simulink model "AOCS_FDIR"  (R2020a)
settings: Solver=ode45  StartTime=0.0  StopTime=86400  FixedStep=1e-4  MaxStep=0.1  RelTol=1e-3  AbsTol=1e-3
undefined symbols (not defined in the file or in its folder): A, A_FEEP, A_FEEP_real, A_mag, CG_real, d_face, Dipole_SC, e0_0, e1_0, e2_0, e3_0, e_max_att, e_max_orb, Env_Drag, Env_J2, Env_Moon, Env_Sun, Env_TGG, Env_TMag, FEEP, g, GNSS, gyr, h_ref, h_RW, h_rw_0, I, I_real, IAU, initial_date_JD, J2, K_det, k_quat, km, m, mag, mu, mu_Moon, mu_Sun, n, n_orbits, q_0, Re, RW1, RW2, RW3, RW4, rx0, ry0, rz0, s, sigma1, sigma2, star, T_friction, th_2_gyr, th_FR_gyr, th_RW, th_SD_gyr_null, th_thruster ... (+10)
libraries: dspstat3 x16, aerolibutil x8, sharedutil x6, sharedtransform x5, vrlib x3, aerolibtransform2 x3, aerolibcelestial x2, aerolibgravity2 x1, dspinverses x1
(part 3 of 3)

== matlab function AOCS_FDIR/Navigation/Orbit Filter/MATLAB Function ==
  data: z input; rk1 output; dt input; sig_r input; sig_v input; vk1 output
function [rk1, vk1]  = Kalman(z, dt, sig_r, sig_v)

persistent xk Pk;

%% State transition matrix
A = [1 0 0 dt 0 0; 
     0 1 0 0 dt 0; 
     0 0 1 0 0 dt; 
     0 0 0 1 0 0; 
     0 0 0 0 1 0; 
     0 0 0 0 0 1];
 
%% Process noise matrix 
G = [dt^2/2 0      0;
     0      dt^2/2 0;
     0      0      dt^2/2;
     dt     0      0;
     0      dt     0;
     0      0      dt];
 
Q = 0.25^2*(G*G');
 
%% Sensor noise covariance matrix
R = [sig_r(1)^2 0 0 0 0 0;
     0 sig_r(2)^2 0 0 0 0;
     0 0 sig_r(3)^2 0 0 0;
     0 0 0 sig_v(1)^2 0 0;
     0 0 0 0 sig_v(2)^2 0;
     0 0 0 0 0 sig_v(3)^2];
 
%% Initialize States and Measurement
if isempty(xk)
    % Initialize states
    xk = z;
    
    % Initialize Covariance Matrix. Farrenkopf’s steady-state analysis
    Pk = R;
    
    % Initialize Measurement
    xk1    = xk;
    rk1 = xk1(1:3);
    vk1 = xk1(4:6);
    
    return;
end

%% Prediction
xk1 = A*xk;
Pk1 = A*Pk*A'+Q;

%% Correction
K   = Pk1/(Pk1+R);
xk1 = xk1 + K*(z-xk1);
Pk1 = (eye(6)-K)*Pk1;

rk1 = xk1(1:3);
vk1 = xk1(4:6);

%% Update
xk = xk1;
Pk = Pk1;

return

== matlab function AOCS_FDIR/Control/Attitude Control/Reaction Wheel Model/Desaturation/MATLAB Function1 ==
  data: us input; T_det output; T_mt input; A_rw input
function T_det = fcn(us, T_mt, A_rw)

delta_u = (A_rw'/(A_rw*A_rw'))*(T_mt-A_rw*us);
T_det   = delta_u;

== matlab function AOCS_FDIR/Navigation/Gyroscope/Gyroscope Model/Artificial Failure/MATLAB Function2 ==
  settings: updateMethod=DISCRETE
  data: t input; flag1 input; flag2 input; flag3 input; in input; out output
function out = fcn(t, flag1, flag2, flag3,in)

persistent frozen
persistent t0

drift = 1e-6;

if isempty(frozen)
    frozen=0;
end

if isempty(t0)
    t0=0;
end

if flag1>0
%% Sudden Death
    out = 0;
elseif flag2>0
%% Frozen Signal
    if frozen == 0
        frozen=in;
        out = in;
    else
        out = frozen;
    end
elseif flag3>0
    %% Drift x
    if t0 == 0
        t0=t;
        out = in;
    else
        out = in + drift*1.37*(t-t0);
    end
else
    out = in;
    frozen = 0;
    t0 = 0;
end

== matlab function AOCS_FDIR/FDIR/Gyroscopes FDIR/Level 1/Diagnosis Frozen Signal/MATLAB Function ==
  settings: updateMethod=DISCRETE
  data: std_1 input; flag_FR_1 output; std_2 input; std_3 input; std_4 input; std_5 input; std_6 input; th_FR_gyr input; win_length input; gyr_rate input; t input; flag_FR_2 output; flag_FR_3 output; flag_FR_4 output; flag_FR_5 output; flag_FR_6 output
function [flag_FR_1,flag_FR_2,flag_FR_3,flag_FR_4,flag_FR_5,flag_FR_6] = fcn(std_1,std_2,std_3,std_4,std_5,std_6,th_FR_gyr, win_length, gyr_rate, t)
%% Define persistent variables
persistent flag1
persistent flag2
persistent flag3
persistent flag4
persistent flag5
persistent flag6

if isempty(flag1)
    flag1 = 0;
end

if isempty(flag2)
    flag2 = 0;
end

if isempty(flag3)
    flag3 = 0;
end

if isempty(flag4)
    flag4 = 0;
end

if isempty(flag5)
    flag5 = 0;
end

if isempty(flag6)
    flag6 = 0;
end

%% Wait to moving std stabilization
if t<win_length*gyr_rate
    flag_FR_1 = flag1;
    flag_FR_2 = flag2;
    flag_FR_3 = flag3;
    flag_FR_4 = flag4;
    flag_FR_5 = flag5;
    flag_FR_6 = flag6;
    return
end

%% Detect the Frozen Condition
if std_1<th_FR_gyr
    flag1 = 1;   
end

if std_2<th_FR_gyr
    flag2 = 1;   
end

if std_3<th_FR_gyr
    flag3 = 1;   
end

if std_4<th_FR_gyr
    flag4 = 1;   
end

if std_5<th_FR_gyr
    flag5 = 1;   
end

if std_6<th_FR_gyr
    flag6 = 1;   
end

%% Create the output
flag_FR_1 = flag1;
flag_FR_2 = flag2;
flag_FR_3 = flag3;
flag_FR_4 = flag4;
flag_FR_5 = flag5;
flag_FR_6 = flag6;

== matlab function AOCS_FDIR/FDIR/Gyroscopes FDIR/Level 1/MATLAB Function ==
  data: flag_SD input; flagLevel1 output; flag_FR input
function flagLevel1 = fcn(flag_SD, flag_FR)
%% Define persistent variables
persistent flag

if isempty(flag)
    flag = zeros(6,1);
end

%% Detect the failure
if flag_SD(1)>0 || flag_FR(1)>0
    flag(1) = 1;
end

if flag_SD(2)>0 || flag_FR(2)>0
    flag(2) = 1;
end

if flag_SD(3)>0 || flag_FR(3)>0
    flag(3) = 1;
end

if flag_SD(4)>0 || flag_FR(4)>0
    flag(4) = 1;
end

if flag_SD(5)>0 || flag_FR(5)>0
    flag(5) = 1;
end

if flag_SD(6)>0 || flag_FR(6)>0
    flag(6) = 1;
end

%% Create the output
flagLevel1 = flag;

== matlab function AOCS_FDIR/Navigation/Gyroscope/Gyroscope Model/Gyroscope Recovery ==
  data: H_in input; H_out output; flagLevel1 input; flagLevel2 input
function H_out = fcn(H_in,flagLevel1,flagLevel2)
%% Switch off (=0) the faulty gyroscopes
% Number 1
if flagLevel1(1) == 0
    if flagLevel2(1) == 0
        switch_m1 = 1;
    else
        switch_m1 = 0;
    end
else
    switch_m1 = 0;
end

% Number 2
if flagLevel1(2) == 0
    if flagLevel2(2) == 0
        switch_m2 = 1;
    else
        switch_m2 = 0;
    end
else
    switch_m2 = 0;
end

% Number 3
if flagLevel1(3) == 0
    if flagLevel2(3) == 0
        switch_m3 = 1;
    else
        switch_m3 = 0;
    end
else
    switch_m3 = 0;
end

% Number 4
if flagLevel1(4) == 0
    if flagLevel2(4) == 0
        switch_m4 = 1;
    else
        switch_m4 = 0;
    end
else
    switch_m4 = 0;
end

% Number 5
if flagLevel1(5) == 0
    if flagLevel2(5) == 0
        switch_m5 = 1;
    else
        switch_m5 = 0;
    end
else
    switch_m5 = 0;
end

% Number 6
if flagLevel1(6) == 0
    if flagLevel2(6) == 0
        switch_m6 = 1;
    else
        switch_m6 = 0;
    end
else
    switch_m6 = 0;
end

%% Final configuration matrix
H_out = [H_in(1,:)*switch_m1;
         H_in(2,:)*switch_m2;
         H_in(3,:)*switch_m3;
         H_in(4,:)*switch_m4;
         H_in(5,:)*switch_m5;
         H_in(6,:)*switch_m6];

== matlab function AOCS_FDIR/Control/Attitude Control/Reaction Wheel Model/Artificial Failure1/MATLAB Function ==
  settings: updateMethod=DISCRETE
  data: in input; h_RW input; T_friction input; out output; flag1 input; flag2 input; flag3 input
function out = fcn(in, h_RW, T_friction, flag1, flag2, flag3)

if flag1>0
%% Motor failure
    out = T_friction*sign(h_RW);
elseif flag2>0
%% Friction failure
    out = in*0.75;
elseif flag3>0
%% Loss of accuracy
    out = in*(1-0.3*randn);
else
    out = in;
end

== matlab function AOCS_FDIR/Navigation/Gyroscope/Gyroscope Model/Isolation Switch off  ==
  data: in input; out output; flagLevel1 input; flagLevel2 input
function out = fcn(in, flagLevel1, flagLevel2)
%% The signal from the faulty gyroscopes must be null
% Number 1
if flagLevel1(1) == 0
    if flagLevel2(1) == 0
        switch_m1 = 1;
    else
        switch_m1 = 0;
    end
else
    switch_m1 = 0;
end

% Number 2
if flagLevel1(2) == 0
    if flagLevel2(2) == 0
        switch_m2 = 1;
    else
        switch_m2 = 0;
    end
else
    switch_m2 = 0;
end

% Number 3
if flagLevel1(3) == 0
    if flagLevel2(3) == 0
        switch_m3 = 1;
    else
        switch_m3 = 0;
    end
else
    switch_m3 = 0;
end

% Number 4
if flagLevel1(4) == 0
    if flagLevel2(4) == 0
        switch_m4 = 1;
    else
        switch_m4 = 0;
    end
else
    switch_m4 = 0;
end

% Number 5
if flagLevel1(5) == 0
    if flagLevel2(5) == 0
        switch_m5 = 1;
    else
        switch_m5 = 0;
    end
else
    switch_m5 = 0;
end

% Number 6
if flagLevel1(6) == 0
    if flagLevel2(6) == 0
        switch_m6 = 1;
    else
        switch_m6 = 0;
    end
else
    switch_m6 = 0;
end

%% Compute output signal
out = [in(1)*switch_m1;
       in(2)*switch_m2;
       in(3)*switch_m3;
       in(4)*switch_m4;
       in(5)*switch_m5;
       in(6)*switch_m6];

== matlab function AOCS_FDIR/FDIR/Gyroscopes FDIR/Level 2/Fault Detection ==
  settings: updateMethod=DISCRETE
  data: flagr1 input; flagm1 output; flagr2 input; flagr3 input; flagr4 input; flagr5 input; flagr6 input; flagr7 input; flagr8 input; flagr9 input; flag input; flagm2 output; flagm3 output; flagm4 output; flagm5 output; flagm6 output
function [flagm1, flagm2, flagm3, flagm4, flagm5, flagm6] = fcn(flagr1, flagr2, flagr3, flagr4, flagr5, flagr6, flagr7, flagr8, flagr9,flag)
%% Define persistent variables
persistent flag1
persistent flag2
persistent flag3
persistent flag4
persistent flag5
persistent flag6

if isempty(flag1)
    flag1=0;
end

if isempty(flag2)
    flag2=0;
end

if isempty(flag3)
    flag3=0;
end

if isempty(flag4)
    flag4=0;
end

if isempty(flag5)
    flag5=0;
end

if isempty(flag6)
    flag6=0;
end

%% Failure dectection
if flag>0
    if flagr1 == 0
        if flagr2 ==1
            if flagr4 ==0
                flag6 = 1;
            elseif flagr4 ==1
                if flagr5 == 0
                    flag3 = 1;
                elseif flagr5 == 1
                    flag3 = 1;
                    flag6 = 1;
                end
            end
        end
    elseif flagr1 == 1
        if flagr2 == 0
            if flagr6 == 0
                flag4 = 1;
            elseif flagr6 == 1
                if flagr7 == 0
                    flag1 = 1;
                elseif flagr7 == 1
                    flag1 = 1;
                    flag4 = 1;
                end
            end
        elseif flagr2 == 1
            if flagr3 == 0
                if flagr4 == 0
                    flag2 = 1;
                elseif flagr4 == 1
                    if flagr5 == 0
                        flag5 = 1;
                    elseif flagr5 == 1
                        flag2 = 1;
                        flag5 = 1;
                    end
                end
            elseif flagr3 == 1
                if flagr7 == 0
                    flag1 = 1;
                    flag3 = 1;
                elseif flagr5 == 0
                    flag3 = 1;
                    flag5 = 1;
                elseif flagr6 == 0
                    flag4 = 1;
                    flag6 = 1;
                elseif flagr4 == 0
                    flag2 = 1;
                    flag6 = 1;
                elseif flagr9 == 0
                    flag1 = 1;
                    flag5 = 1;
                elseif flagr8 == 0
                    flag2 = 1;
                    flag4 = 1;
                end
            end
        end
    end
end


%% Assign the output
flagm1 = flag1;
flagm2 = flag2;
flagm3 = flag3;
flagm4 = flag4;
flagm5 = flag5;
flagm6 = flag6;

== matlab function AOCS_FDIR/Navigation/Gyroscope/Gyroscope Model/Artificial Failure/MATLAB Function1 ==
  settings: updateMethod=DISCRETE
  data: t input; flag1 input; flag2 input; flag3 input; in input; out output
function out = fcn(t, flag1, flag2, flag3,in)

persistent frozen
persistent t0

drift = 1e-6;

if isempty(frozen)
    frozen=0;
end

if isempty(t0)
    t0=0;
end

if flag1>0
%% Sudden Death
    out = 0;
elseif flag2>0
%% Frozen Signal
    if frozen == 0
        frozen=in;
        out = in;
    else
        out = frozen;
    end
elseif flag3>0
    %% Drift x
    if t0 == 0
        t0=t;
        out = in;
    else
        out = in + drift*1.15*(t-t0);
    end
else
    out = in;
    frozen = 0;
    t0 = 0;
end

== matlab function AOCS_FDIR/Control/Attitude Control/Reaction Wheel Model/Artificial Failure2/MATLAB Function ==
  settings: updateMethod=DISCRETE
  data: in input; h_RW input; T_friction input; out output; flag1 input; flag2 input; flag3 input
function out = fcn(in, h_RW, T_friction, flag1, flag2, flag3)

if flag1>0
%% Motor failure
    out = T_friction*sign(h_RW);
elseif flag2>0
%% Friction failure
    out = in*0.75;
elseif flag3>0
%% Loss of accuracy
    out = in*(1-0.3*randn);
else
    out = in;
end

== matlab function AOCS_FDIR/Control/Attitude Control/Reaction Wheel Model/Isolation2/MATLAB Function ==
  data: T_in input; T_out output; stop input; h_RW input; T_friction input; flagRW input
function T_out = fcn(T_in, stop, h_RW, T_friction, flagRW)

if flagRW>0
    if stop>0
        T_out = 0;
    else
        T_out = T_friction*sign(h_RW);
    end
else
    T_out = T_in;
end

== matlab function AOCS_FDIR/Control/Attitude Control/Reaction Wheel Model/Artificial Failure3/MATLAB Function ==
  settings: updateMethod=DISCRETE
  data: in input; h_RW input; T_friction input; out output; flag1 input; flag2 input; flag3 input
function out = fcn(in, h_RW, T_friction, flag1, flag2, flag3)

if flag1>0
%% Motor failure
    out = T_friction*sign(h_RW);
elseif flag2>0
%% Friction failure
    out = in*0.75;
elseif flag3>0
%% Loss of accuracy
    out = in*(1-0.3*randn);
else
    out = in;
end

== matlab function AOCS_FDIR/FDIR/Gyroscopes FDIR/Level 2/Residuals Generator ==
  data: w_gyr input; r1 output; r2 output; r3 output; r4 output; r5 output; r6 output; r7 output; r8 output; r9 output
function [r1,r2,r3,r4,r5,r6,r7,r8,r9] = fcn(w_gyr)
%% Measurements from gyroscopes
m1 = w_gyr(1);
m2 = w_gyr(2);
m3 = w_gyr(3);
m4 = w_gyr(4);
m5 = w_gyr(5);
m6 = w_gyr(6);

%% Residuals for detection
r1 = (m1+m4) - (m2+m5);
r2 = (m2+m5) - (m3+m6);
r3 = (m3+m6) - (m1+m4);

%% Residuals for isolation
r4 = 2*(m1+m3+m5) - 3*(m1+m4);
r5 = 2*(m2+m4+m6) - 3*(m1+m4);
r6 = 2*(m1+m3+m5) - 3*(m2+m5);
r7 = 2*(m2+m4+m6) - 3*(m2+m5);
r8 = 2*(m1+m3+m5) - 3*(m3+m6);
r9 = 2*(m2+m4+m6) - 3*(m3+m6);

== matlab function AOCS_FDIR/FDIR/Reaction Wheels FDIR/RW Diagnosis/Diagnosis Reaction Wheels ==
  settings: updateMethod=DISCRETE
  data: r_RW1 input; flagRW1 output; r_RW2 input; r_RW3 input; r_RW4 input; t input; RW_rate input; win_length input; flagRW2 output; flagRW3 output; flagRW4 output; th_RW input
function [flagRW1, flagRW2, flagRW3, flagRW4] = fcn(r_RW1, r_RW2, r_RW3, r_RW4, t, RW_rate, win_length,th_RW)

persistent flag

if t<2*win_length*RW_rate
    flagRW1 = 0;
    flagRW2 = 0;
    flagRW3 = 0;
    flagRW4 = 0;
    return
end

if isempty(flag)
    flag = zeros(4,1);
end

if r_RW1>th_RW
    flag(1) = 1;
end

if r_RW2>th_RW
    flag(2) = 1;
end

if r_RW3>th_RW
    flag(3) = 1;
end

if r_RW4>th_RW
    flag(4) = 1;
end

flagRW1 = flag(1);
flagRW2 = flag(2);
flagRW3 = flag(3);
flagRW4 = flag(4);

== matlab function AOCS_FDIR/Control/Attitude Control/Reaction Wheel Model/Isolation1/MATLAB Function ==
  data: T_in input; T_out output; stop input; h_RW input; T_friction input; flagRW input
function T_out = fcn(T_in, stop, h_RW, T_friction, flagRW)

if flagRW>0
    if stop>0
        T_out = 0;
    else
        T_out = T_friction*sign(h_RW);
    end
else
    T_out = T_in;
end

== matlab function AOCS_FDIR/Visualization/COE/MATLAB Function ==
  data: R input; a output; V input; e output; i output; RA output; w output; TA output
function [a, e, i, RA, w, TA] = sv2coe(R,V)
%-------------------------------------------------------------------------
% This function computes the classical orbital elements (coe)
% from the state vector (R,V).
%
% mu - gravitational parameter (mˆ3/sˆ2)
% R - position vector in ECI (m)
% V - velocity vector in ECI (m)
% r, v - the moduli of R and V
% vr - radial velocity component (m/s)
% H - the angular momentum vector (mˆ2/s)
% h - the moduli of H (mˆ2/s)
% i - inclination of the orbit (rad)
% N - the node line vector (mˆ2/s)
% n - the moduli of N
% cp - cross product of N and R
% RA - right ascension of the ascending node (rad)
% E - eccentricity vector
% e - eccentricity (moduli of E)
% eps - a small number below which the eccentricity is
% considered to be zero
% w - argument of perigee (rad)
% TA - true anomaly (rad)
% a - semimajor axis (m)
% coe - vector of orbital elements [a, e, i, RA, w, TA]
%
% ------------------------------------------------------------------------
%% Inputs
mu = 3.986004418e14;
eps = 1.e-10;

r = norm(R);
v = norm(V);
vr = dot(R,V)/r;

H = cross(R,V);
h = norm(H);

%% Inclination
i = acosd(H(3)/h);

%% Node line
N = cross([0 0 1],H);
n = norm(N);

%% Right Ascension
if n ~= 0
    RA = acosd(N(1)/n);
    if N(2) < 0
        RA = 360 - RA;
    end
else
    RA= 0;                 % No defined asceding node (Equatorial orbit)
end

%% Eccentricity
E = 1/mu*((v^2 - mu/r)*R - r*vr*V);
e = norm(E);

%% Argument of periapsis
% To avoid numerical errors
d_N_E=dot(N,E)/n/e;
if d_N_E>1 
    d_N_E = 1;
elseif d_N_E<-1
    d_N_E = -1;
end

if n ~= 0
    if e > eps
        w = acosd(d_N_E);
        if E(3) < 0
            w = 360 - w;
        end
    else
        w = 0;             % No defined periapsis (Circular orbit)    
    end
else
    w = 0;                 % No defined ascending node (Equatorial orbits)
end


%% True anomaly
% To avoid numerical errors
d_E_R=dot(E,R)/e/r;
if d_E_R>1 
    d_E_R = 1;
elseif d_E_R<-1
    d_E_R = -1;
end

d_N_R=dot(N,R)/n/r;
if d_N_R>1 
    d_N_R = 1;
elseif d_N_R<-1
    d_N_R = -1;
end

if e > eps
    TA = norm(acosd(d_E_R));
    if vr < 0
        TA = 360 - TA;
    end
else
    cp = cross(N,R);
    if cp(3) >= 0
        TA = acosd(d_N_R);
    else
        TA = 360 - acosd(d_N_R);
    end
end

%% Semimajor axis
a = h^2/mu/(1 - e^2);

== matlab function AOCS_FDIR/Control/Attitude Control/Reaction Wheel Allocation/Recovery ==
  data: RW1 input; A_rw output; RW2 input; RW3 input; RW4 input; flagRW1 input; flagRW2 input; flagRW3 input; flagRW4 input
function A_rw = fcn(RW1, RW2, RW3, RW4, flagRW1, flagRW2, flagRW3, flagRW4)
%% Switch off (=0) the faulty wheels
% Wheel 1
if flagRW1>0
    flag1 = 0;
else
    flag1 = 1;
end

% Wheel 2
if flagRW2>0
    flag2 = 0;
else
    flag2 = 1;
end

% Wheel 3
if flagRW3>0
    flag3 = 0;
else
    flag3 = 1;
end

% Wheel 4
if flagRW4>0
    flag4 = 0;
else
    flag4 = 1;
end

%% Reconfigure configuration matrix
A_rw = [RW1*flag1,RW2*flag2,RW3*flag3,RW4*flag4];

== matlab function AOCS_FDIR/Control/Attitude Control/Reaction Wheel Model/Desaturation/Recovery ==
  data: RW1 input; A_rw output; RW2 input; RW3 input; RW4 input; flagRW1 input; flagRW2 input; flagRW3 input; flagRW4 input
function A_rw = fcn(RW1, RW2, RW3, RW4, flagRW1, flagRW2, flagRW3, flagRW4)
%% Switch off (=0) the faulty wheels
% Wheel 1
if flagRW1>0
    flag1 = 0;
else
    flag1 = 1;
end

% Wheel 2
if flagRW2>0
    flag2 = 0;
else
    flag2 = 1;
end

% Wheel 3
if flagRW3>0
    flag3 = 0;
else
    flag3 = 1;
end

% Wheel 4
if flagRW4>0
    flag4 = 0;
else
    flag4 = 1;
end

%% Reconfigure configuration matrix
A_rw = [RW1*flag1,RW2*flag2,RW3*flag3,RW4*flag4];

== matlab function AOCS_FDIR/FDIR/Gyroscopes FDIR/Level 2/Evaluation ==
  data: S1 input; flagr1 output; S2 input; S3 input; S4 input; S5 input; S6 input; S7 input; S8 input; S9 input; win_length input; th input; flagr2 output; flagr3 output; flagr4 output; flagr5 output; flagr6 output; flagr7 output; flagr8 output; flagr9 output; flag output
function [flagr1, flagr2, flagr3, flagr4, flagr5, flagr6, flagr7,flagr8,flagr9,flag] = fcn(S1, S2, S3, S4, S5, S6, S7,S8,S9, win_length, th)
%% Define persistent variables
persistent state
persistent count

if isempty(count)
    state =zeros(9,2);
end

if isempty(count)
    count=0;
end

%% Evaluation of thresholds
if S1>th
    flagr1 = 1;
else
    flagr1 = 0;
end

if S2>th
    flagr2 = 1;
else
    flagr2 = 0;
end

if S3>th
    flagr3 = 1;
else
    flagr3 = 0;
end

if S4>th
    flagr4 = 1;
else
    flagr4 = 0;
end

if S5>th
    flagr5 = 1;
else
    flagr5 = 0;
end

if S6>th
    flagr6 = 1;
else
    flagr6 = 0;
end

if S7>th
    flagr7 = 1;
else
    flagr7 = 0;
end

if S8>th
    flagr8 = 1;
else
    flagr8 = 0;
end

if S9>th
    flagr9 = 1;
else
    flagr9 = 0;
end

%% Wait for stabilization of all residuals
for i=2
    state(:,i-1) = state(:,i);
end

state(1,2) = flagr1;
state(2,2) = flagr2;
state(3,2) = flagr3;
state(4,2) = flagr4;
state(5,2) = flagr5;
state(6,2) = flagr6;
state(7,2) = flagr7;
state(8,2) = flagr8;
state(9,2) = flagr9;

for i=1:9
    if state(i,1)~= state(i,2)
        count = 0;
    end
end

if flagr1>0 || flagr2>0 || flagr3>0
    count = count+1;
else
    count = 0;
end

if count>0.5*win_length
    flag = 1;
else
    flag =0;
end

== matlab function AOCS_FDIR/Navigation/Gyroscope/Gyroscope Model/Artificial Failure/MATLAB Function3 ==
  settings: updateMethod=DISCRETE
  data: t input; flag1 input; flag2 input; flag3 input; in input; out output
function out = fcn(t, flag1, flag2, flag3,in)

persistent frozen
persistent t0

drift = 1e-6;

if isempty(frozen)
    frozen=0;
end

if isempty(t0)
    t0=0;
end

if flag1>0
%% Sudden Death
    out = 0;
elseif flag2>0
%% Frozen Signal
    if frozen == 0
        frozen=in;
        out = in;
    else
        out = frozen;
    end
elseif flag3>0
    %% Drift x
    if t0 == 0
        t0=t;
        out = in;
    else
        out = in + drift*0.87*(t-t0);
    end
else
    out = in;
    frozen = 0;
    t0 = 0;
end

== matlab function AOCS_FDIR/Navigation/Gyroscope/Gyroscope Model/Artificial Failure/MATLAB Function4 ==
  settings: updateMethod=DISCRETE
  data: t input; flag1 input; flag2 input; flag3 input; in input; out output
function out = fcn(t, flag1, flag2, flag3,in)

persistent frozen
persistent t0

drift = 1e-6;

if isempty(frozen)
    frozen=0;
end

if isempty(t0)
    t0=0;
end

if flag1>0
%% Sudden Death
    out = 0;
elseif flag2>0
%% Frozen Signal
    if frozen == 0
        frozen=in;
        out = in;
    else
        out = frozen;
    end
elseif flag3>0
    %% Drift x
    if t0 == 0
        t0=t;
        out = in;
    else
        out = in + drift*(t-t0);
    end
else
    out = in;
    frozen = 0;
    t0 = 0;
end

== matlab function AOCS_FDIR/Navigation/Gyroscope/Gyroscope Model/Artificial Failure/MATLAB Function5 ==
  settings: updateMethod=DISCRETE
  data: t input; flag1 input; flag2 input; flag3 input; in input; out output
function out = fcn(t, flag1, flag2, flag3,in)

persistent frozen
persistent t0

drift = 1e-6;

if isempty(frozen)
    frozen=0;
end

if isempty(t0)
    t0=0;
end

if flag1>0
%% Sudden Death
    out = 0;
elseif flag2>0
%% Frozen Signal
    if frozen == 0
        frozen=in;
        out = in;
    else
        out = frozen;
    end
elseif flag3>0
    %% Drift x
    if t0 == 0
        t0=t;
        out = in;
    else
        out = in + drift*0.9*(t-t0);
    end
else
    out = in;
    frozen = 0;
    t0 = 0;
end

== matlab function AOCS_FDIR/Navigation/Gyroscope/Gyroscope Model/Artificial Failure/MATLAB Function6 ==
  settings: updateMethod=DISCRETE
  data: t input; flag1 input; flag2 input; flag3 input; in input; out output
function out = fcn(t, flag1, flag2, flag3,in)

persistent frozen
persistent t0

drift = 1e-6;

if isempty(frozen)
    frozen=0;
end

if isempty(t0)
    t0=0;
end

if flag1>0
%% Sudden Death
    out = 0;
elseif flag2>0
%% Frozen Signal
    if frozen == 0
        frozen=in;
        out = in;
    else
        out = frozen;
    end
elseif flag3>0
    %% Drift x
    if t0 == 0
        t0=t;
        out = in;
    else
        out = in + drift*0.66*(t-t0);
    end
else
    out = in;
    frozen = 0;
    t0 = 0;
end

== matlab function AOCS_FDIR/Control/Attitude Control/Reaction Wheel Model/Isolation3/MATLAB Function ==
  data: T_in input; T_out output; stop input; h_RW input; T_friction input; flagRW input
function T_out = fcn(T_in, stop, h_RW, T_friction, flagRW)

if flagRW>0
    if stop>0
        T_out = 0;
    else
        T_out = T_friction*sign(h_RW);
    end
else
    T_out = T_in;
end

== matlab function AOCS_FDIR/Control/Attitude Control/Reaction Wheel Model/Artificial Failure4/MATLAB Function ==
  settings: updateMethod=DISCRETE
  data: in input; h_RW input; T_friction input; out output; flag1 input; flag2 input; flag3 input
function out = fcn(in, h_RW, T_friction, flag1, flag2, flag3)

if flag1>0
%% Motor failure
    out = T_friction*sign(h_RW);
elseif flag2>0
%% Friction failure
    out = in*0.75;
elseif flag3>0
%% Loss of accuracy
    out = in*(1-0.3*randn);
else
    out = in;
end

== matlab function AOCS_FDIR/Control/Attitude Control/Reaction Wheel Model/Isolation4/MATLAB Function ==
  data: T_in input; T_out output; stop input; h_RW input; T_friction input; flagRW input
function T_out = fcn(T_in, stop, h_RW, T_friction, flagRW)

if flagRW>0
    if stop>0
        T_out = 0;
    else
        T_out = T_friction*sign(h_RW);
    end
else
    T_out = T_in;
end

== matlab function AOCS_FDIR/Visualization/COE/MATLAB Function1 ==
  data: R input; a output; V input; e output; i output; RA output; w output; TA output
function [a, e, i, RA, w, TA] = sv2coe(R,V)
%-------------------------------------------------------------------------
% This function computes the classical orbital elements (coe)
% from the state vector (R,V).
%
% mu - gravitational parameter (mˆ3/sˆ2)
% R - position vector in ECI (m)
% V - velocity vector in ECI (m)
% r, v - the moduli of R and V
% vr - radial velocity component (m/s)
% H - the angular momentum vector (mˆ2/s)
% h - the moduli of H (mˆ2/s)
% i - inclination of the orbit (rad)
% N - the node line vector (mˆ2/s)
% n - the moduli of N
% cp - cross product of N and R
% RA - right ascension of the ascending node (rad)
% E - eccentricity vector
% e - eccentricity (moduli of E)
% eps - a small number below which the eccentricity is
% considered to be zero
% w - argument of perigee (rad)
% TA - true anomaly (rad)
% a - semimajor axis (m)
% coe - vector of orbital elements [a, e, i, RA, w, TA]
%
% ------------------------------------------------------------------------
%% Inputs
mu = 3.986004418e14;
eps = 1.e-10;

r = norm(R);
v = norm(V);
vr = dot(R,V)/r;

H = cross(R,V);
h = norm(H);

%% Inclination
i = acosd(H(3)/h);

%% Node line
N = cross([0 0 1],H);
n = norm(N);

%% Right Ascension
if n ~= 0
    RA = acosd(N(1)/n);
    if N(2) < 0
        RA = 360 - RA;
    end
else
    RA= 0;                 % No defined asceding node (Equatorial orbit)
end

%% Eccentricity
E = 1/mu*((v^2 - mu/r)*R - r*vr*V);
e = norm(E);

%% Argument of periapsis
% To avoid numerical errors
d_N_E=dot(N,E)/n/e;
if d_N_E>1 
    d_N_E = 1;
elseif d_N_E<-1
    d_N_E = -1;
end

if n ~= 0
    if e > eps
        w = acosd(d_N_E);
        if E(3) < 0
            w = 360 - w;
        end
    else
        w = 0;             % No defined periapsis (Circular orbit)    
    end
else
    w = 0;                 % No defined ascending node (Equatorial orbits)
end


%% True anomaly
% To avoid numerical errors
d_E_R=dot(E,R)/e/r;
if d_E_R>1 
    d_E_R = 1;
elseif d_E_R<-1
    d_E_R = -1;
end

d_N_R=dot(N,R)/n/r;
if d_N_R>1 
    d_N_R = 1;
elseif d_N_R<-1
    d_N_R = -1;
end

if e > eps
    TA = norm(acosd(d_E_R));
    if vr < 0
        TA = 360 - TA;
    end
else
    cp = cross(N,R);
    if cp(3) >= 0
        TA = acosd(d_N_R);
    else
        TA = 360 - acosd(d_N_R);
    end
end

%% Semimajor axis
a = h^2/mu/(1 - e^2);

== matlab function AOCS_FDIR/FDIR/Gyroscopes FDIR/Level 1/Diagnosis Sudden Death/Diagnosis Sudden Death Gyroscope ==
  data: dm1 input; flag_SD_1 output; m1 input; dm2 input; m2 input; dm3 input; m3 input; dm4 input; m4 input; dm5 input; m5 input; dm6 input; m6 input; flag_SD_2 output; flag_SD_3 output; flag_SD_4 output; flag_SD_5 output; flag_SD_6 output; th_SD_gyr_null input
function [flag_SD_1,flag_SD_2,flag_SD_3,flag_SD_4,flag_SD_5,flag_SD_6] = fcn(dm1,m1,dm2,m2,dm3,m3,dm4,m4,dm5,m5,dm6,m6,th_SD_gyr_null)
%% Define persistent variables
persistent flag1
persistent flag2
persistent flag3
persistent flag4
persistent flag5
persistent flag6

if isempty(flag1)
    flag1 = 0;
end

if isempty(flag2)
    flag2 = 0;
end

if isempty(flag3)
    flag3 = 0;
end

if isempty(flag4)
    flag4 = 0;
end

if isempty(flag5)
    flag5 = 0;
end

if isempty(flag6)
    flag6 = 0;
end

%% Detect the Sudden Condition
if dm1>0 && abs(m1)<th_SD_gyr_null
    flag1 = 1;
end

if dm2>0 && abs(m2)<th_SD_gyr_null
    flag2 = 1;
end

if dm3>0 && abs(m3)<th_SD_gyr_null
    flag3 = 1;
end

if dm4>0 && abs(m4)<th_SD_gyr_null
    flag4 = 1;
end

if dm5>0 && abs(m5)<th_SD_gyr_null
    flag5 = 1;
end

if dm6>0 && abs(m6)<th_SD_gyr_null
    flag6 = 1;
end

%% Create the output
flag_SD_1 = flag1;
flag_SD_2 = flag2;
flag_SD_3 = flag3;
flag_SD_4 = flag4;
flag_SD_5 = flag5;
flag_SD_6 = flag6;

== matlab function AOCS_FDIR/Control/Orbit Control/Thruster Model/Artificial Failure/MATLAB Function ==
  data: in input; out output; flag1 input; flag2 input; flag3 input; flag4 input; flag5 input; flag6 input; flag7 input; flag8 input
function out = fcn(in,flag1,flag2,flag3,flag4,flag5,flag6,flag7,flag8)

out = in.*[flag1;flag2;flag3;flag4;flag5;flag6;flag7;flag8];

== matlab function AOCS_FDIR/Control/Orbit Control/Thruster Allocation/Isolation & Recovery ==
  data: A_FEEP input; y output; flag input
function y = fcn(A_FEEP, flag)

y =[A_FEEP(:,1)*(1-flag(1)), A_FEEP(:,2)*(1-flag(2)), A_FEEP(:,3)*(1-flag(3)), A_FEEP(:,4)*(1-flag(4)), A_FEEP(:,5)*(1-flag(5)), A_FEEP(:,6)*(1-flag(6)), A_FEEP(:,7)*(1-flag(7)), A_FEEP(:,8)*(1-flag(8))];

== matlab function AOCS_FDIR/FDIR/Gyroscopes FDIR/Level 2/GLR Test ==
  settings: updateMethod=DISCRETE
  data: r1 input; S1 output; r2 input; r3 input; r4 input; r5 input; r6 input; r7 input; r8 input; r9 input; win_length input; sigma1 input; sigma2 input; S2 output; S3 output; S4 output; S5 output; S6 output; S7 output; t input; gyr_rate input; S8 output; S9 output
function [S1,S2,S3,S4,S5,S6,S7,S8,S9] = fcn(r1,r2,r3,r4,r5,r6,r7,r8,r9,win_length,sigma1,sigma2,t,gyr_rate)
%% Define window length
N = win_length;

%% Define persistent variable to compute GLR test
persistent s

if isempty(s)
    s = zeros(9,N);
end

for i=2:N
    s(1,i-1) = s(1,i);
    s(2,i-1) = s(2,i);
    s(3,i-1) = s(3,i);
    s(4,i-1) = s(4,i);
    s(5,i-1) = s(5,i);
    s(6,i-1) = s(6,i);
    s(7,i-1) = s(7,i);
    s(8,i-1) = s(8,i);
    s(9,i-1) = s(9,i);
end

s(1,N) = r1;
s(2,N) = r2;
s(3,N) = r3;
s(4,N) = r4;
s(5,N) = r5;
s(6,N) = r6;
s(7,N) = r7;
s(8,N) = r8;
s(9,N) = r9;

%% Compute GLR test for each residual
if t<win_length*gyr_rate                                                    % Wait for stabilization of statistics variables
    S1 = 0;
    S2 = 0;
    S3 = 0;
    S4 = 0;
    S5 = 0;
    S6 = 0;
    S7 = 0;
    S8 = 0;
    S9 = 0;
else  
    S1 = sum((s(1,:)-0))^2/(2*sigma1^2*N);
    S2 = sum((s(2,:)-0))^2/(2*sigma1^2*N);
    S3 = sum((s(3,:)-0))^2/(2*sigma1^2*N);
    S4 = sum((s(4,:)-0))^2/(2*sigma2^2*N);
    S5 = sum((s(5,:)-0))^2/(2*sigma2^2*N);
    S6 = sum((s(6,:)-0))^2/(2*sigma2^2*N);
    S7 = sum((s(7,:)-0))^2/(2*sigma2^2*N);
    S8 = sum((s(8,:)-0))^2/(2*sigma2^2*N);
    S9 = sum((s(9,:)-0))^2/(2*sigma2^2*N);
end

== matlab function AOCS_FDIR/FDIR/Thrusters FDIR/Thruster Diagnosis/MATLAB Function7 ==
  settings: updateMethod=DISCRETE
  data: r input; win_length input; sigma input; S1 output
function S1  = fcn(r, win_length,sigma)
%% Define window length
N = win_length;

%% Define persistent variable for GLR test computation
persistent s1

if isempty(s1)
    s1 = zeros(1,N);
end

for i=2:N
    s1(1,i-1) = s1(1,i);
end

s1(1,N) = r;

%% GLR test applied to the mean value(=0)
S1 = sum((s1-0))^2/(2*sigma^2*N);

== matlab function AOCS_FDIR/FDIR/Thrusters FDIR/Thruster Diagnosis/Residual Calculation ==
  settings: updateMethod=DISCRETE
  data: I input; q input; Pk1_EKF input; u input; y input; rate input; r output
function r  = fcn(I, q,  Pk1_EKF, u, y, rate)

persistent xk Pk;

%% State transition matrix
w=y;

Ixx = I(1);
Iyy = I(5);
Izz = I(9);

A = [0, -(Izz-Iyy)*w(3)/Ixx, -(Izz-Iyy)*w(2)/Ixx;
     -(Ixx-Izz)*w(3)/Iyy, 0, -(Ixx-Izz)*w(1)/Iyy;
     -(Iyy-Ixx)*w(2)/Izz, -(Iyy-Ixx)*w(1)/Izz, 0];

A = expm(A*rate);
 
%% Control matrix
B = rate*inv(I);

%% Measurement matrix
C = eye(3);

%% Process noise matrix 
Q = eye(3)*q;
 
%% Sensor noise covariance matrix
R = Pk1_EKF;
 
if isempty(xk)
    %% Initialize States and Measurement
    % Initialize states
    xk = y;
    
    % Initialize Covariance Matrix
    Pk = R;
    
    % Initialize residual
    r = y-C*xk;
return
end

%% Prediction
xk1 = A*xk+B*u;
Pk1 = A*Pk*A'+Q;

%% Kalman Gain
K = Pk1*C'/(C*Pk1*C'+R);

%% Correction
xk1 = xk1+K*(y-C*xk1);
Pk1 = (eye(3)-K*C)*Pk*(eye(3)-K*C)'+K*R*K';

%% Residual
r = y-C*xk1;

%% Next step
xk = xk1;
Pk = Pk1;

== matlab function AOCS_FDIR/FDIR/Thrusters FDIR/Thruster Diagnosis/MATLAB Function10 ==
  settings: updateMethod=DISCRETE
  data: r input; win_length input; sigma input; S1 output
function S1  = fcn(r, win_length,sigma)
%% Define window length
N = win_length;

%% Define persistent variable for GLR test computation
persistent s1

if isempty(s1)
    s1 = zeros(1,N);
end

for i=2:N
    s1(1,i-1) = s1(1,i);
end

s1(1,N) = r;

%% GLR test applied to the mean value(=0)
S1 = sum((s1-0))^2/(2*sigma^2*N);

== matlab function AOCS_FDIR/FDIR/Thrusters FDIR/Thruster Diagnosis/MATLAB Function8 ==
  settings: updateMethod=DISCRETE
  data: r input; win_length input; sigma input; S1 output
function S1  = fcn(r, win_length,sigma)
%% Define window length
N = win_length;

%% Define persistent variable for GLR test computation
persistent s1

if isempty(s1)
    s1 = zeros(1,N);
end

for i=2:N
    s1(1,i-1) = s1(1,i);
end

s1(1,N) = r;

%% GLR test applied to the mean value(=0)
S1 = sum((s1-0))^2/(2*sigma^2*N);

== matlab function AOCS_FDIR/FDIR/Thrusters FDIR/Thruster Diagnosis/MATLAB Function9 ==
  data: u input; y output
function y = fcn(u)

y = u(4:6,4:6);

== matlab function AOCS_FDIR/FDIR/Thrusters FDIR/Thruster Diagnosis/MATLAB Function ==
  settings: updateMethod=DISCRETE
  data: S1 input; flagt1 output; mean1 input; S2 input; mean2 input; S3 input; mean3 input; flagt2 output; flagt3 output; flagt4 output; flagt5 output; flagt6 output; flagt7 output; flagt8 output; th_thruster input; firing input; n_thruster output; t input
function [flagt1, flagt2, flagt3, flagt4, flagt5, flagt6, flagt7, flagt8, n_thruster] = fcn(S1,mean1,S2,mean2,S3,mean3,th_thruster, firing,t)
%% Define persistent flag
persistent flag1
persistent flag2
persistent flag3
persistent flag4
persistent flag5
persistent flag6
persistent flag7
persistent flag8
persistent t0

if isempty(flag1)
    flag1 = 0;
    flag2 = 0;
    flag3 = 0;
    flag4 = 0;
    flag5 = 0;
    flag6 = 0;
    flag7 = 0;
    flag8 = 0;
    t0 = 0;
end

%% Define mean acumalated in memory
persistent m1
persistent m2
persistent m3
N = 500;

if isempty(m1)
    m1 = zeros(1,N);
    m2 = zeros(1,N);
    m3 = zeros(1,N);
end

for i=2:N
    m1(1,i-1) = m1(1,i);
    m2(1,i-1) = m2(1,i);
    m3(1,i-1) = m3(1,i);
end

m1(1,N) = mean1;
m2(1,N) = mean2;
m3(1,N) = mean3;

%% Find the faulty thruster

if firing >0 && t > (500+t0) 
    if S1>th_thruster || S2>th_thruster || S3>th_thruster
        d1 = m1(end)-m1(1);
        d2 = m2(end)-m2(1);
        d3 = m3(end)-m3(1);
        t0 = t;
        if d1>0
            if d2>0
                if d3>0
                    flag8 = 1;
                elseif d3<0
                    flag2 = 1;
                end
            elseif d2<0
                if d3>0
                    flag7 = 1;
                elseif d3<0
                    flag1 = 1;
                end
            end
        elseif d1<0
            if d2>0
                if d3>0
                    flag6 = 1;
                elseif d3<0
                    flag4 = 1;
                end
            elseif d2<0
                if d3>0
                    flag5 = 1;
                elseif d3<0
                    flag3 = 1;
                end
            end
        end
    end
end

%% Assign the outputs
flagt1 = flag1;
flagt2 = flag2;
flagt3 = flag3;
flagt4 = flag4;
flagt5 = flag5;
flagt6 = flag6;
flagt7 = flag7;
flagt8 = flag8;

n_thruster = 8 - (flagt1+ flagt2+ flagt3+ flagt4+ flagt5+ flagt6+ flagt7+ flagt8);

== matlab function AOCS_FDIR/Dynamics/Environmet/Atmospheric drag/Atmospheric Density ==
  data: h input; rho output
function rho = Exponential_Atm_Model(h)
%% Initialization
rho = 0;

%% Parameters of the model
h_0   = [0; 25; 30; 35; 40; 45; 50; 55; 60; 65; 70; 75; 80; 85; 90; 95; 100; 110; 120; 130; 140; 150; 160; 180; 200; 250; 300; 350; 400; 450; 500; 600; 700; 800; 900; 1000];
rho_0 = [1.225; 3.899e-2; 1.774e-2; 8.279e-3; 3.972e-3; 1.995e-3; 1.057e-3; 5.821e-4; 3.206e-4; 1.718e-4; 8.770e-5; 4.178e-5; 1.905e-5; 8.337e-6; 3.396e-6; 1.343e-6; 5.297e-7; 9.661e-8; 2.438e-8; 8.484e-9; 3.845e-9; 2.070e-9; 1.224e-9; 5.464e-10; 2.789e-10; 7.248e-11; 2.418e-11; 9.158e-12; 3.725e-12; 1.585e-12; 6.967e-13; 1.454e-13; 3.614e-14; 1.170e-14; 5.245e-15; 3.019e-15];
H     = [8.44; 6.49; 6.75; 7.07; 7.47; 7.83; 7.95; 7.73; 7.29; 6.81; 6.33; 6.00; 5.70; 5.41; 5.38; 5.74; 6.15; 8.06; 11.6; 16.1; 20.6; 24.6; 26.3; 33.2; 38.5; 46.9; 52.5; 56.4; 59.4; 62.2; 65.8; 79; 109; 164; 225; 268];

%% Compute the density as a function of altitude
if h<=h_0(2)
    rho = rho_0(1)*exp(-(h-h_0(1))/H(1));
elseif h>h_0(end)
    rho = rho_0(end)*exp(-(h-h_0(end)/H(end)));
else
    for i=2:(length(h_0)-1)
        if h>h_0(i) && h<=h_0(i+1)
            rho = rho_0(i)*exp(-(h-h_0(i))/H(i));
        end
    end
end

end

== matlab function AOCS_FDIR/Dynamics/Environmet/Atmospheric drag/MATLAB Function ==
  data: v_rel_ECI input; a_Drag output; v_rel_b input; rho input; m input; T_Drag output; n input; A input; d_face input
function [a_Drag, T_Drag] = fcn(v_rel_ECI, v_rel_b, rho, m, n, A, d_face)
%% Initialization
a_Drag = zeros(3,1);
T_Drag = zeros(3,1);

%% Compute incidence and CD
incidence = n*(v_rel_b/norm(v_rel_b));
CD = 4*incidence.^3;

%% Calculation of total drag and torque
for i=1:size(n,1)
    if incidence(i)>0
        a_Drag = a_Drag + (-0.5*rho*CD(i)*A(i)*incidence(i)/m*...
            norm(v_rel_ECI)*v_rel_ECI);
        T_Drag = T_Drag + cross(d_face(i)*n(i,:),(-0.5*rho*CD(i)*A(i)*incidence(i)*...
            norm(v_rel_b)*v_rel_b))';
    else
        continue
    end
end

== matlab function AOCS_FDIR/Visualization/3D Orbit/3D Orbit Plot ==
  settings: updateMethod=DISCRETE
  data: x input; v input; DCM input; time input
function fcn(x,v,DCM,time)

persistent initialize;
persistent pc1;
persistent pc2;
persistent pc3;
persistent pc4;
persistent pc5;
persistent pc6;
persistent pc7;
persistent pc8;
persistent pc9;
persistent pc10;
persistent pc11;
persistent pc12;
persistent pc13;
persistent pc14;
persistent th;
persistent th1;
persistent th2;
persistent th3;
persistent time0;
persistent globe;
persistent orbit;
% persistent i_LVLH;
% persistent j_LVLH;
% persistent k_LVLH;

coder.extrinsic('patch');
coder.extrinsic('delete')
coder.extrinsic('earth_example')
coder.extrinsic('mArrow3')
coder.extrinsic('cylinder2P')
coder.extrinsic('ellipsoid')
coder.extrinsic('imread')
coder.extrinsic('rotate')
coder.extrinsic('animatedline')
coder.extrinsic('addpoints')

if isempty(initialize)
    figure(1)
    axes('Units', 'normalized', 'Position', [0 0 1 1])
    hold on
    
    % Customize the window
    set(gcf,'Menubar','none','Name','3D Orbit', ...
        'NumberTitle','off','Position',[0,0,825,840], ...
        'Color',[0 0 0]);
    
    % Plot the Earth in the correct position
    npanels = 180;
    erad    = 6378137;
    prad    = 6356752.31424518;
    [x, y, z] = ellipsoid(0, 0, 0, erad, erad, prad, npanels);
    
    image_file = 'ModifiedBlueMarble.jpg';
    
    globe=surf(x, y, -1*z, 'FaceColor', 'none', 'EdgeColor', 0.5*[1 1 1]);
    
    cdata = imread(image_file);
    set(globe, 'FaceColor', 'texturemap', 'CData', cdata, 'FaceAlpha', 1, 'EdgeColor', 'none');
    material(globe,'dull')
    
    set(gcf,'Color','k');
    
    % Plot ECI frame
    b = 9000000;
    mArrow3([0 0 0],b*[1 0 0]','color','yellow','stemWidth',1e5);
    mArrow3([0 0 0],b*[0 1 0]','color','yellow','stemWidth',1e5);
    mArrow3([0 0 0],b*[0 0 1]','color','yellow','stemWidth',1e5);
    text(b,0,0.15*b,'x','Color','y')
    text(0,b,0.15*b,'y','Color','y')
    text(0,0.1*b,b,'z','Color','y')
    
    % Customize the view 
    view(135,20);
    light('Position',[2,0.5,0.5]);
    lighting gouraud; 
    axis off;
    axis equal;
    axis([-10000000 10000000 -10000000 10000000 -10000000 10000000])
 
    initialize = 1;
    pc1        = patch(1e6*[0 0 1 1],1e6*[0 1 1 0],1e6*[1 1 1 1],'b');
    pc2        = patch(1e6*[0 0 1 1],1e6*[0 1 1 0],1e6*[1 1 1 1],'b');
    pc3        = patch(1e6*[0 0 1 1],1e6*[0 1 1 0],1e6*[1 1 1 1],'b');
    pc4        = patch(1e6*[0 0 1 1],1e6*[0 1 1 0],1e6*[1 1 1 1],'b');
    pc5        = patch(1e6*[0 0 1 1],1e6*[0 1 1 0],1e6*[1 1 1 1],'b');
    pc6        = patch(1e6*[0 0 1 1],1e6*[0 1 1 0],1e6*[1 1 1 1],'b');
    pc7        = patch(1e6*[0 0 1 1],1e6*[0 1 1 0],1e6*[1 1 1 1],'b');
    pc8        = patch(1e6*[0 0 1 1],1e6*[0 1 1 0],1e6*[1 1 1 1],'b');
    pc9        = patch(1e6*[0 0 1 1],1e6*[0 1 1 0],1e6*[1 1 1 1],'b');
    pc10       = patch(1e6*[0 0 1 1],1e6*[0 1 1 0],1e6*[1 1 1 1],'b');
    pc11       = patch(1e6*[0 0 1 1],1e6*[0 1 1 0],1e6*[1 1 1 1],'b');
    pc12       = patch(1e6*[0 0 1 1],1e6*[0 1 1 0],1e6*[1 1 1 1],'b');
    pc13       = patch(1e6*[0 0 1 1],1e6*[0 1 1 0],1e6*[1 1 1 1],'b');
    pc14       = patch(1e6*[0 0 1 1],1e6*[0 1 1 0],1e6*[1 1 1 1],'b');
    th         = patch(1e6*[0 0 1 1],1e6*[0 1 1 0],1e6*[1 1 1 1],'b');
    th1        = patch(1e6*[0 0 1 1],1e6*[0 1 1 0],1e6*[1 1 1 1],'b');
    th2        = patch(1e6*[0 0 1 1],1e6*[0 1 1 0],1e6*[1 1 1 1],'b');
    th3        = patch(1e6*[0 0 1 1],1e6*[0 1 1 0],1e6*[1 1 1 1],'b');
    
    rotate(globe,[0 0 -1],22, [0 0 0]);
    orbit = animatedline('Color','r');
    time0 = 0;
    
else
    figure(1)
    rotate(globe,[0 0 1],(time-time0)*360/86400, [0 0 0]);
    
    ll = 5e5;
    %czoom = 13;
    
    delete(pc1)
    delete(pc2)
    delete(pc3)
    delete(pc4)
    delete(pc5)
    delete(pc6)
    delete(pc7)
    delete(pc8)
    delete(pc9)
    delete(pc10)
    delete(pc11)
    delete(pc12)
    delete(pc13)
    delete(pc14)
    delete(th)
    delete(th1)
    delete(th2)
    delete(th3)
    
    ii = x/sqrt(x(1)^2+x(2)^2+x(3)^2);
    jj = v/sqrt(v(1)^2+v(2)^2+v(3)^2);
    
    % Plot the orbit
    addpoints(orbit,x(1),x(2),x(3));
    
    %plot3(x(1),x(2),x(3),'ro','MarkerSize',2)
    %plot3(x_des(1),x_des(2),x_des(3),'bo','MarkerSize',1)
    
    % Satellite
    
    vpc1  = [ll*[0.5 0.5 0.5 0.5];2*ll*[-0.5 -0.5 0.5 0.5]; ll*[-0.5 0.5 0.5 -0.5]];
    vpc2  = [ll*[-0.5 -0.5 -0.5 -0.5];2*ll*[-0.5 -0.5 0.5 0.5];ll*[-0.5 0.5 0.5 -0.5]];
    vI1   = 0.6*DCM'*vpc1;
    vI2   = 0.6*DCM'*vpc2;
    
    pc1 = patch(x(1)+vI1(1,:),x(2)+vI1(2,:),x(3)+vI1(3,:),'blue');
    pc2 = patch(x(1)+vI2(1,:),x(2)+vI2(2,:),x(3)+vI2(3,:),'blue');
    %
    
    vpc1  = [ll*[0.5 0.5 -0.5 -0.5];2*ll*[-0.5 0.5  0.5 -0.5];ll*[-0.5 -0.5 -0.5 -0.5]];
    vpc2  = [ll*[0.5 0.5 -0.5 -0.5];2*ll*[-0.5 0.5  0.5 -0.5];ll*[ 0.5  0.5  0.5  0.5]];
    vI1   = 0.6*DCM'*vpc1;
    vI2   = 0.6*DCM'*vpc2;
    
    pc3 = patch(x(1)+vI1(1,:),x(2)+vI1(2,:),x(3)+vI1(3,:),'blue');
    pc4 = patch(x(1)+vI2(1,:),x(2)+vI2(2,:),x(3)+vI2(3,:),'blue');
    %
    vpc1  = [ll*[0.5 0.5 -0.5 -0.5];2*ll*[0.5 0.5  0.5 0.5];ll*[ 0.5 -0.5 -0.5 0.5]];
    vpc2  = [ll*[0.5 0.5 -0.5 -0.5];2*ll*[-0.5 -0.5  -0.5 -0.5];ll*[ 0.5  -0.5  -0.5  0.5]];
    vI1   = 0.6*DCM'*vpc1;
    vI2   = 0.6*DCM'*vpc2;
    
    pc5 = patch(x(1)+vI1(1,:),x(2)+vI1(2,:),x(3)+vI1(3,:),'blue');
    pc6 = patch(x(1)+vI2(1,:),x(2)+vI2(2,:),x(3)+vI2(3,:),'blue');
    
    % Solar Panel 
%     vB1  = [ll*[0 0 0 0];ll*[1 3 3 1]; ll*[ -0.5 -0.5 +0.5 0.5]];
%     vB2  = [ll*[0 0 0 0];ll*[-1 -3 -3 -1];ll*[ -0.5 -0.5  +0.5 0.5]];
%     vI1   = 0.6*DCM'*vB1;
%     vI2   = 0.6*DCM'*vB2;
    
    %pc7 = patch(x(1)+vI1(1,:),x(2)+vI1(2,:),x(3)+vI1(3,:),'white');
    %pc8 = patch(x(1)+vI2(1,:),x(2)+vI2(2,:),x(3)+vI2(3,:),'white');
    
%     % THRUSTER
%     r   = ll/4;
%     r1  = (ll*[-0.5, -0.5, -0.5] + ll*[-0.5, 0.5, 0.5])/2;
%     vr1 = x + DCM'*r1';
%     vr2 = vr1 - ll/3*DCM(1,:)';
%     
%     [X, Y, Z] = cylinder2P(r, 20,vr1',vr2');
%         th=surf(X,Y,Z,'facecolor','white');
%     [X, Y, Z] = cylinder2P(ll/5, 40,vr1',(vr2- ll/8*DCM(1,:)')');
%         th1=surf(X,Y,Z,'facecolor','red');
%     [X, Y, Z] = cylinder2P(ll/6, 40,vr1',(vr2-ll/5*DCM(1,:)')');
%         th2=surf(X,Y,Z,'facecolor','red');
%     [X, Y, Z] = cylinder2P(ll/7, 40,vr1',(vr2- ll/3*DCM(1,:)')');
%         th3=surf(X,Y,Z,'facecolor','red');
    
    % LVLH
    k_LVLH = -x/norm(x);
    j_LVLH = -cross(x,v)/norm(cross(x,v));
    i_LVLH = cross(j_LVLH,k_LVLH);
    pc9  = mArrow3(x,x + ll*1.8*i_LVLH,'color','yellow','stemWidth',ll/20);
    pc10 = mArrow3(x,x + ll*1.8*j_LVLH,'color','yellow','stemWidth',ll/20);
    pc11 = mArrow3(x,x + ll*1.8*k_LVLH,'color','yellow','stemWidth',ll/20);
    
    % BODY FRAME
    pc12 = mArrow3(x,x + ll*1.8*DCM(1,:)','color','cyan','stemWidth',ll/20);
    pc13 = mArrow3(x,x + ll*1.8*DCM(2,:)','color','red','stemWidth',ll/20);
    pc14 = mArrow3(x,x + ll*1.8*DCM(3,:)','color','green','stemWidth',ll/20);
    
    %xlim([-20e7 20e7])
    %ylim([-20e7 20e7])
    %zlim([-20e7 20e7])
    
    material(pc1,'dull')
    material(pc2,'dull')
    material(pc3,'dull')
    material(pc4,'dull')
    material(pc5,'dull')
    material(pc6,'dull')
    material(pc7,'metal')
    material(pc8,'metal')
    material(th,'metal')
    
    %campos([x(1)+czoom*ll*ii(1),x(2)+czoom*ll*ii(2),x(3)+czoom*ll*ii(3)]) % vista segun r
    %campos([x(1),x(2),x(3)+czoom*ll]) % vista de arriba
    % segun vector velocidad
    %campos([x(1)+czoom*ll*jj(1),x(2)+czoom*ll*jj(2),x(3)+czoom*ll*jj(3)])
    
    
    %camtarget([x(1),x(2),x(3)])
    %camtarget([0,0,0])
   
    %camva(80)
    %earth_example
    
    time0 = time;
    
    drawnow
end

== matlab function AOCS_FDIR/Visualization/Groundtrack/Groundtrack ==
  settings: updateMethod=DISCRETE
  data: lat input; lon input
function fcn(lat, lon)

persistent initialize;
persistent groundtrack;
persistent lon0;
persistent sat1;
persistent sat2;
persistent sat3;
persistent sat4;

coder.extrinsic('animatedline')
coder.extrinsic('addpoints')
coder.extrinsic('imread')
coder.extrinsic('imagesc')
coder.extrinsic('delete')
coder.extrinsic('patch')
coder.extrinsic('line')

if isempty(initialize)
     figure(2)
    % Customize the window
    set(gcf,'Menubar','none','Name','Groundtrack', ...
        'NumberTitle','off','Position',[825,42,710,355], ...
        'Color',[1 1 1]);

    % Plot the worldmap
    img = imread('ModifiedBlueMarble.jpg');
    
    min_x = -180;
    max_x = 180;
    min_y = -90;
    max_y = 90;
    
    imagesc([min_x max_x], [min_y max_y], flipud(img));
    lon0 = lon;
    
    % Customize the view
    set(gca,'Ydir','default','GridColor','k','GridAlpha',0.4,...
        'XTick',-180:30:180,'YTick',-90:30:90)
    axis([min_x,max_x,min_y, max_y])
    grid on;
    
    sat1        = patch([1 0 -1 0]*2.75+lon,[0 1 0 -1]*2.75+lat,'k');
    sat2        = line([-0.75 0.75]*2.75+lon,[0.75,-0.75]*2.75+lat,'Color','k');
    sat3        = patch([-1 -0.5 -2 -2.5]*2.75+lon, [0.5 1 2.5 2]*2.75+lat,'white');
    sat4        = patch([-1 -0.5 -2 -2.5]*-2.75+lon, [0.5 1 2.5 2]*-2.75+lat,'white');
    initialize  = 1;
    groundtrack = animatedline('Color','r');
    
else     
    figure(2)
    delete(sat1)
    delete(sat2)
    delete(sat3)
    delete(sat4)
    
    if sind(lon0)*sind(lon)<=0
        groundtrack = animatedline('Color','r');
        addpoints(groundtrack,lon,lat);
    else
        addpoints(groundtrack,lon,lat);
    end
    
    sat1 = patch([1 0 -1 0]*2.5+lon,[0 1 0 -1]*2.5+lat,'k');
    sat2 = line([-0.75 0.75]*2.5+lon,[0.75,-0.75]*2.5+lat,'Color','k');
    sat3 = patch([-1 -0.5 -1.5 -2]*2.5+lon, [0.5 1 2 1.5]*2.5+lat,'white');
    sat4 = patch([-1 -0.5 -1.5 -2]*-2.5+lon, [0.5 1 2 1.5]*-2.5+lat,'white');
      
    lon0 = lon;
    drawnow
end
